simulink model "manitius_ex2_simu_R2016a"  (R2016a)
settings: Solver=VariableStepAuto  SolverMode=SingleTasking  StartTime=0.0  StopTime=Tsim  RelTol=1e-3
values from neighbouring files (symbols this model uses):
  a = 2    [manitius_ex2_code.m]
  A1z = dssP1.A    [manitius_ex1_code.m]    (also in manitius_ex2_code.m)
  b1 = 1    [manitius_ex2_code.m]
  B1z = dssP1.B    [manitius_ex1_code.m]    (also in manitius_ex2_code.m)
  C1z = dssP1.C    [manitius_ex1_code.m]    (also in manitius_ex2_code.m)
  f = (p-a)/ba    [manitius_ex2_code.m]
  h = 2    [manitius_ex1_code.m]    (also in manitius_ex2_code.m)
  N = block.DialogPrm(5).Data    [IntW.m]    (also in manitius_ex1_code.m = 1000; manitius_ex2_code.m = 2000)
undefined symbols (not defined in the file or in its folder): Ad1, Bd1, Cd1, Dd1, KSoma1, Q1, tal1
settings Model: Creator=Vasco  LastModifiedBy=Vasco
settings DebuggingCC: UnconnectedInputMsg=none  UnconnectedOutputMsg=none  UnconnectedLineMsg=none  SFUnexpectedBacktrackingDiag=error  SFNoUnconditionalDefaultTransitionDiag=error
settings ModelReferenceCC: EnableRefExpFcnMdlSchedulingChecks=off
settings SFSimCC: SimUseLocalCustomCode=on
settings RTWCC: Description=Generic Real-Time Target  RTWUseLocalCustomCode=on
settings GRTTargetCC: TargetLangStandard=C99 (ISO)
settings ConfigComp: CovMetricSettings=dwe  CovSaveCumulativeToWorkspaceVar=off  CovSaveSingleToWorkspaceVar=off  CovExternalEMLEnable=on

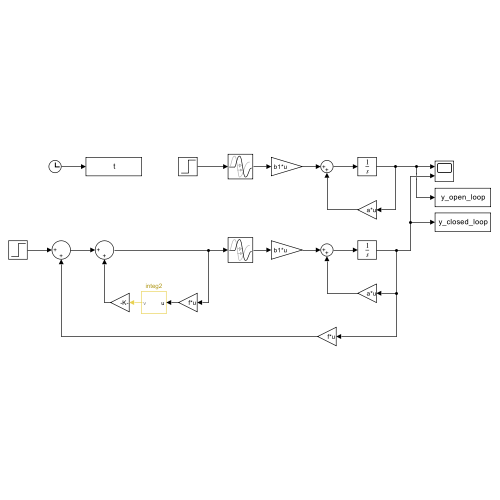
[thumbnail: Simulink's stored preview of the top-level diagram]
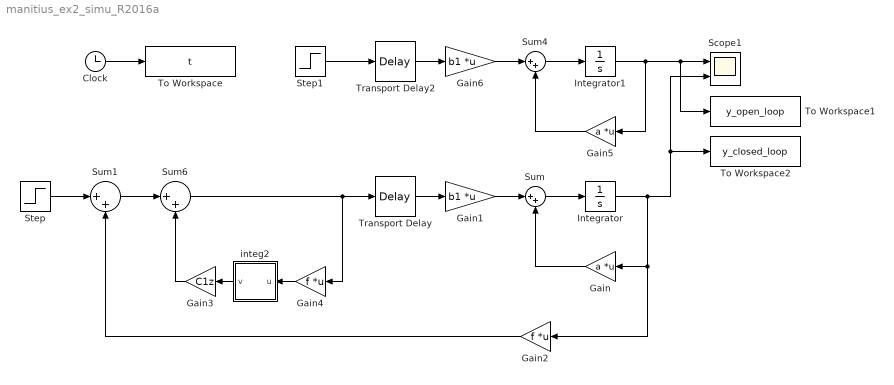
== system manitius_ex2_simu_R2016a ==
  Clock : Clock
  Gain : Gain  Gain=a  Multiplication=Matrix(K*u)
  Gain1 : Gain  Gain=b1  Multiplication=Matrix(K*u)
  Gain2 : Gain  Gain=f  Multiplication=Matrix(K*u)
  Gain3 : Gain  Gain=C1z
  Gain4 : Gain  Gain=f  Multiplication=Matrix(K*u)
  Gain5 : Gain  Gain=a  Multiplication=Matrix(K*u)
  Gain6 : Gain  Gain=b1  Multiplication=Matrix(K*u)
  Integrator : Integrator
  Integrator1 : Integrator
  Scope1 : Scope  NumInputPorts=2
  Step : Step  Time=0  SampleTime=0
  Step1 : Step  Time=0  SampleTime=0
  Sum{,1,4,6} (4 alike) : Sum  Inputs=|++
  To Workspace : ToWorkspace  VariableName=t  SampleTime=-1
  To Workspace1 : ToWorkspace  VariableName=y_open_loop  SampleTime=-1
  To Workspace2 : ToWorkspace  VariableName=y_closed_loop  SampleTime=-1
  Transport Delay : TransportDelay  DelayTime=h
  Transport Delay2 : TransportDelay  DelayTime=h
  integ2 : Subsystem
  wires:
  Sum/1 -> Integrator/1
  Gain/1 -> Sum/2
  Gain2/1 -> Sum1/2
  Step/1 -> Sum1/1
  Transport Delay/1 -> Gain1/1
  Gain1/1 -> Sum/1
  Integrator/1 -> To Workspace2/1, Scope1/2, Gain/1, Gain2/1
  Sum1/1 -> Sum6/1
  Gain3/1 -> Sum6/2
  Sum6/1 -> Transport Delay/1, Gain4/1
  Gain4/1 -> integ2/1(u)
  Sum4/1 -> Integrator1/1
  Gain6/1 -> Sum4/1
  Gain5/1 -> Sum4/2
  Step1/1 -> Transport Delay2/1
  Transport Delay2/1 -> Gain6/1
  Integrator1/1 -> Gain5/1, To Workspace1/1, Scope1/1
  Clock/1 -> To Workspace/1
  integ2/1(v) -> Gain3/1

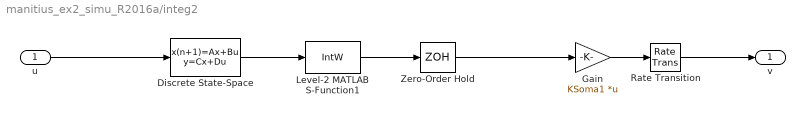
== system manitius_ex2_simu_R2016a/integ2 ==
  u : Inport
  Discrete State-Space : DiscreteStateSpace  A=Ad1  B=Bd1  C=Cd1  D=Dd1  SampleTime=tal1
  Gain : Gain  Gain=KSoma1  Multiplication=Matrix(K*u)
  Level-2 MATLAB S-Function1 : M-S-Function  FunctionName=IntW  Parameters=tal1,A1z,B1z,Q1,N
  Rate Transition : RateTransition
  Zero-Order Hold : ZeroOrderHold  SampleTime=tal1
  v : Outport
  wires:
  Rate Transition/1 -> v/1
  u/1 -> Discrete State-Space/1
  Gain/1 -> Rate Transition/1
  Zero-Order Hold/1 -> Gain/1
  Discrete State-Space/1 -> Level-2 MATLAB S-Function1/1
  Level-2 MATLAB S-Function1/1 -> Zero-Order Hold/1
